simulink model "validate_engine_state"  (R2015a)
settings: Solver=ode45  StartTime=0.0  StopTime=10.0  RelTol=1e-3
undefined symbols (not defined in the file): sigbuilder_block
libraries: MotoHawk_lib x1
settings Model: NumberOfSteps=5  Creator=Piyush  LastModifiedBy=Piyush

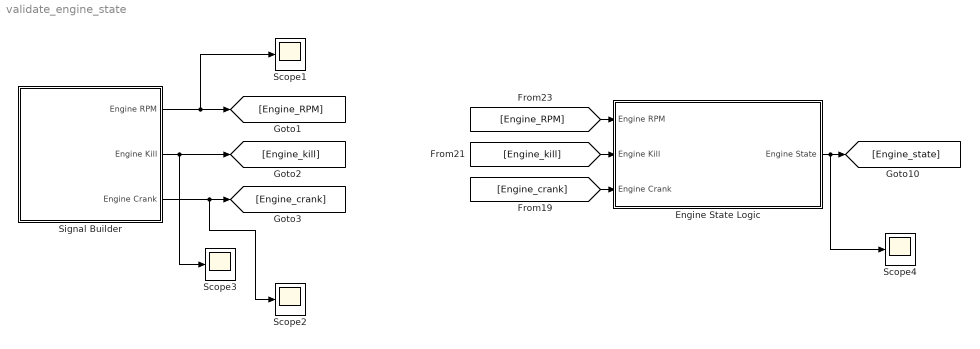
== system validate_engine_state ==
  Engine State Logic : Subsystem
  Scope{1..4} (4 alike) : Scope
      Scope2 settings: SaveName=ScopeData2
      Scope3 settings: SaveName=ScopeData3
  Signal Builder : Subsystem  Tag=STV Subsys  LoadFcn=sigbuilder_block('load',[0.75 30.75 510.75 481.5 ]);  StartFcn=sigbuilder_block('start');  StopFcn=sigbuilder_block('stop');  ClipboardFcn=sigbuilder_block('clipboard');  mask(Sigbuilder block){}
      mask help: Simulink:masks:SigbuilderBlock_MD
      mask init:
      | if ~strcmp(get_param(bdroot(gcbh),'SimulationStatus'),'stopped') tuvar = sigbuilder_block('maskInit'); end
      settings: CopyFcn=sigbuilder_block('copy');  DeleteFcn=sigbuilder_block('delete');  ModelCloseFcn=sigbuilder_block('modelClose');  PreSaveFcn=sigbuilder_block('preSave');  PauseFcn=sigbuilder_block('pause');  ContinueFcn=sigbuilder_block('continue');  NameChangeFcn=sigbuilder_block('namechange');  OpenFcn=sigbuilder_block('open',[437.6 199.2 550.4 400 ]);  CloseFcn=sigbuilder_block('close');
      mask Display: plot(0, 0, 100, 100,[2, 2, 32, 32, 2], [68, 8, 8, 68, 68],[32, 2], [38, 38], [32, 19, 2],[53, 60, 44], [32, 17, 17, 2],[16, 16, 31, 31]);txt = getActiveGroup(gcbh);text(2, 100, txt,'verticalAlignment', 'top');
  wires:
  Engine State Logic/1(Engine State) -> Scope4/1, [Engine_state]
  [Engine_kill] -> Engine State Logic/2(Engine Kill)
  [Engine_RPM] -> Engine State Logic/1(Engine RPM)
  [Engine_crank] -> Engine State Logic/3(Engine Crank)
  Signal Builder/1(Engine RPM) -> Scope1/1, [Engine_RPM]
  Signal Builder/2(Engine Kill) -> Scope3/1, [Engine_kill]
  Signal Builder/3(Engine Crank) -> Scope2/1, [Engine_crank]

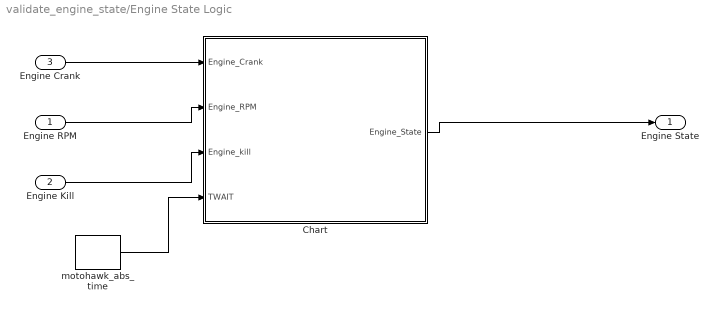
== system validate_engine_state/Engine State Logic ==
  Engine RPM : Inport
  Engine Kill : Inport  Port=2
  Engine Crank : Inport  Port=3
  Chart : Stateflow chart  TreatAsAtomicUnit=on
  motohawk_abs_time : MotoHawk_lib/Extra Development Blocks/motohawk_abs_time  mode=Seconds (double)  width=64 bit
  Engine State : Outport
  wires:
  Engine Crank/1 -> Chart/1(Engine_Crank)
  Engine Kill/1 -> Chart/3(Engine_kill)
  Engine RPM/1 -> Chart/2(Engine_RPM)
  Chart/1(Engine_State) -> Engine State/1
  motohawk_abs_time/1 -> Chart/4(TWAIT)

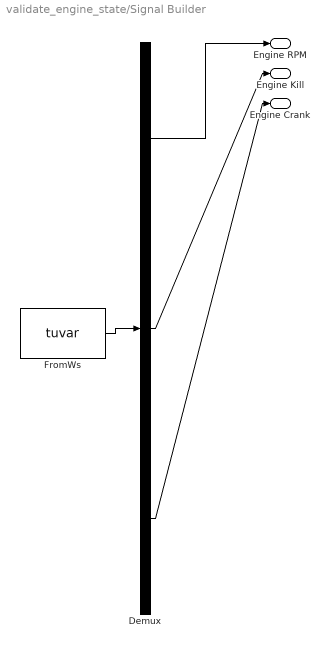
== system validate_engine_state/Signal Builder ==
  Demux : Demux  Tag=STV Demux  Outputs=3
  FromWs : FromWorkspace  Tag=STV FromWs  VariableName=tuvar  SampleTime=0
      SigBuilderData=|
      | common.afterFinalStr = 'Extrapolate'
      | common.sampleTime = 0
      | dataSet.timeRange = [0 10]
      | dataSet.name = 'Group 1'
      | sbobj.Groups.Name = 'Group 1'
      | sbobj.Groups.Signals(1).Name = 'Engine RPM'
      | sbobj.Groups.Signals(1).XData = [0 1.01 1.01 1.99 3.06 6 6 10]
      | sbobj.Groups.Signals(1).YData = [0 0 1 1 870 870 0 0]
      | sbobj.Groups.Signals(2).Name = 'Engine Kill'
      | sbobj.Groups.Signals(2).XData = [0 1.14 1.14 2 2 7.44 7.44 10]
      | sbobj.Groups.Signals(2).YData = [1 1 0 0 1 1 0 0]
      | sbobj.Groups.Signals(3).Name = 'Engine Crank'
      | sbobj.Groups.Signals(3).XData = [0 2.94 2.94 3.96 3.96 10]
      | sbobj.Groups.Signals(3).YData = [0 0 1 1 0 0]
  Engine RPM : Outport  Tag=STV Outport
  Engine Kill : Outport  Tag=STV Outport  Port=2
  Engine Crank : Outport  Tag=STV Outport  Port=3
  wires:
  Demux/1 -> Engine RPM/1
  FromWs/1 -> Demux/1
  Demux/2 -> Engine Kill/1
  Demux/3 -> Engine Crank/1

== stateflow chart validate_engine_state/Engine State Logic/Chart ==
  state EngineCrank
    en: Time_stamp = TWAIT;
    during:Engine_State=2;
  state EngineOff
    during:Engine_State=1;
  state EngineStartFailSate
    during:Engine_State=5;
  state EngineOn
    en: Time_stamp = TWAIT;
    during:Engine_State=4;
  state EngineWarm_up
    en: Time_stamp = TWAIT;
    during: Engine_State=3;
  (default) -> EngineOff
  EngineOff -> EngineCrank : [Engine_Crank==1]
  EngineCrank -> EngineStartFailSate [order 2] : [Engine_RPM<=800&&TWAIT>(Time_stamp+1)]
  EngineCrank -> EngineWarm_up [order 1] : [Engine_RPM>800&&TWAIT>Time_stamp+0.6]
  EngineStartFailSate -> EngineOff
  EngineOn -> EngineOff : [Engine_RPM<50||Engine_kill==1]
  EngineWarm_up -> EngineStartFailSate [order 2] : [Engine_RPM<500 && TWAIT>Time_stamp+1]
  EngineWarm_up -> EngineOn [order 1] : [Engine_RPM>=500&&TWAIT>Time_stamp+1]
  data: Engine_Crank input; Engine_RPM input; Engine_kill input; Engine_State output; TWAIT input; Time_stamp local
